simulink model "kepler_basic_2021b"  (R2021b)
settings: Solver=ode4  StartTime=0.0  StopTime=6000  FixedStep=0.01  RelTol=1e-3
(part 2 of 2)

== matlab function kepler_basic_2021b/[Mode3] Basic Kepler Propagate/MATLAB Function ==
  data: kepel input; statvec output
function statvec  = kepel_statvec (kepel)
%  [statvec] = kepel_statvec (kepel)
%	The function kepel_statvec transforms the keplerian
%	elements kepel into the corresponding state vector in
%	the same reference system.
%
% Input:
%	kepel
% 		vector containing the keplerian elements:
%		(1) - semimajor axis of the orbit in meters.
%		(2) - eccentricity.
%		(3) - inclinatsion in radians.
%		(4) - right ascension of ascending node in radians.
%		(5) - argument of perigee in radians.
%		(6) - mean anomaly in radians.
% Output:
%	statvec
%  		state vector in meters and meters/second.
%
% Authors:
%	Helio K. Kuga;
%	Valder M. Medeiros;
%	Valdemir Carrara		february/80		version 1.0
%	Valdemir Carrara		july 2005		(C version)
%   Valdemir Carrara            March/09        Matlab

EARTH_GRAVITY	= 3.9860064e+14;		% Earth's gravitational constant (m**3/s**2)

a    = kepel(1);	% semi-major axis
exc  = kepel(2);	% eccentricity

c1   = sqrt(1. - exc*exc);

%     rotation matrix

orb2iner = rotmaz(-kepel(4))*rotmax(-kepel(3))*rotmaz(-kepel(5));

%     Kepler's equation

E    = kepler(kepel(6), exc);

sE   = sin(E);
cE   = cos(E);
c3   = sqrt(EARTH_GRAVITY/a)/(1. - exc*cE);

%     state vector

statvec = [[a*(cE - exc), a*c1*sE, 0]*orb2iner', [-c3*sE, c1*c3*cE, 0]*orb2iner'];

end

function [rot_mat] = rotmax (angle)
% [rot_mat] = rotmax (angle)
%   To obtain the rotation matrix around the X axis given the
%   rotation angle.
% inputs:
%   angle
%       rotation angle, in radians.
% outputs:
%   rot_mat
%       rotation matrix (3, 3)
%

% Valdemir Carrara, Sep, 1998

coan    =  cos(angle);
sian    =  sin(angle);

rot_mat =  [1, 0, 0; 0, coan, sian; 0, -sian, coan];

end

function [rot_mat] = rotmay (angle)
% [rot_mat] = rotmay (angle)
%   To obtain the rotation matrix around the Y axis given the
%   rotation angle.
% inputs:
%   angle
%       rotation angle, in radians.
% outputs:
%   rot_mat
%       rotation matrix (3, 3)
%

% Valdemir Carrara, Sep, 1998


coan    =  cos(angle);
sian    =  sin(angle);

rot_mat =  [coan, 0, -sian; 0, 1, 0; sian, 0, coan];

end

function [rot_mat] = rotmaz (angle)
% [rot_mat] = rotmaz (angle)
%   To obtain the rotation matrix around the Z axis given the
%   rotation angle.
% inputs:
%   angle
%       rotation angle, in radians.
% outputs:
%   rot_mat
%       rotation matrix (3, 3)
%

% Valdemir Carrara, Sep, 1998

coan    =  cos(angle);
sian    =  sin(angle);

rot_mat =  [coan, sian, 0; -sian, coan, 0; 0, 0, 1];
end

function [eccentric] = kepler (mean_anomaly, eccentricity)
% [eccentric] = kepler (mean_anomaly, eccentricity)
%	The subroutine kepler finds a solution to the
%	kepler's equation.
%
% Input:
%	mean_anomaly
%		mean anomaly in radians.
%	eccentricity
%		eccentricity.
%
% Output:
%	eccentric
%		eccentric anomaly in radians.
%
% Authors:
%	Valder M. de Medeiros		june/81		version 2.0
%	Valdemir Carrara			july 2005	(C version)
%   Valdemir Carrara            March/09        Matlab

exc2    = eccentricity*eccentricity;
am1     = mod (mean_anomaly, 2*pi);
am2     = am1 + am1;
am3     = am1 + am2;
shoot   = am1 + eccentricity*(1. - 0.125*exc2)*sin(am1) + ...
		0.5*exc2*(sin(am2) + 0.75*eccentricity*sin(am3));
shoot   = mod (shoot, 2*pi);

e1      = 1.0;
ic      = 0;

while ((abs(e1) > 1.e-12) && (ic <= 10)) 
	e1    = (shoot - am1 - eccentricity*sin(shoot)) / ...
			(1.0 - eccentricity*cos(shoot));
    shoot = shoot - e1;
    ic    = ic + 1;
end

if (ic >= 10)
    disp ('warning ** subroutine kepler did not converge in 10 iterations');
end

eccentric = shoot;


end

== matlab function kepler_basic_2021b/[Mode4] Propat vs Kepler:Twobody Equation Integral Comparison/Kepler Propagate ==
  data: initial_condition input; dfdt output
function dfdt  = eq_propagate(initial_condition)
% Lectures_TwoBodyProblem.pdf
% 우주시스템입문 - 도미타 노부유키 eq(7.8) p136
% https://en.wikipedia.org/wiki/Standard_gravitational_parameter
u  = 3.9860064e+14; % earth gravitional parameter
Re = 6378137;      % earth radius [m]

dfdt = zeros(size(initial_condition));

% x=x
% x1=dx/dt
% dx1/dt = d^2(x)/dt

x1 = initial_condition(4); % x1 = dx/dt
y1 = initial_condition(5); % y1 = dy/dt
z1 = initial_condition(6); % z1 = dz/dt
x  = initial_condition(1); % x
y  = initial_condition(2); % y
z  = initial_condition(3); % z

r=sqrt(x^2+y^2+z^2);

% % %   Keplar Motion Equatnion
% % %  => r_dd + u/(r^3)r_ = 0 => r_dd = -u/(r^3)r_
dfdt(1) = x1;
dfdt(2) = y1;
dfdt(3) = z1;
dfdt(4) = -u*x/(r^3);
dfdt(5) = -u*y/(r^3);
dfdt(6) = -u*z/(r^3);

end

== matlab function kepler_basic_2021b/[Mode4] Propat vs Kepler:Twobody Equation Integral Comparison/MATLAB Function2 ==
  data: kepel input; statvec output
function statvec  = kepel_statvec (kepel)
%  [statvec] = kepel_statvec (kepel)
%	The function kepel_statvec transforms the keplerian
%	elements kepel into the corresponding state vector in
%	the same reference system.
%
% Input:
%	kepel
% 		vector containing the keplerian elements:
%		(1) - semimajor axis of the orbit in meters.
%		(2) - eccentricity.
%		(3) - inclinatsion in radians.
%		(4) - right ascension of ascending node in radians.
%		(5) - argument of perigee in radians.
%		(6) - mean anomaly in radians.
% Output:
%	statvec
%  		state vector in meters and meters/second.
%
% Authors:
%	Helio K. Kuga;
%	Valder M. Medeiros;
%	Valdemir Carrara		february/80		version 1.0
%	Valdemir Carrara		july 2005		(C version)
%   Valdemir Carrara            March/09        Matlab

EARTH_GRAVITY	= 3.9860064e+14;		% Earth's gravitational constant (m**3/s**2)

a    = kepel(1);	% semi-major axis
exc  = kepel(2);	% eccentricity

c1   = sqrt(1. - exc*exc);

%     rotation matrix

orb2iner = rotmaz(-kepel(4))*rotmax(-kepel(3))*rotmaz(-kepel(5));

%     Kepler's equation

E    = kepler(kepel(6), exc);

sE   = sin(E);
cE   = cos(E);
c3   = sqrt(EARTH_GRAVITY/a)/(1. - exc*cE);

%     state vector

statvec = [[a*(cE - exc), a*c1*sE, 0]*orb2iner', [-c3*sE, c1*c3*cE, 0]*orb2iner'];

end

function [rot_mat] = rotmax (angle)
% [rot_mat] = rotmax (angle)
%   To obtain the rotation matrix around the X axis given the
%   rotation angle.
% inputs:
%   angle
%       rotation angle, in radians.
% outputs:
%   rot_mat
%       rotation matrix (3, 3)
%

% Valdemir Carrara, Sep, 1998

coan    =  cos(angle);
sian    =  sin(angle);

rot_mat =  [1, 0, 0; 0, coan, sian; 0, -sian, coan];

end

function [rot_mat] = rotmay (angle)
% [rot_mat] = rotmay (angle)
%   To obtain the rotation matrix around the Y axis given the
%   rotation angle.
% inputs:
%   angle
%       rotation angle, in radians.
% outputs:
%   rot_mat
%       rotation matrix (3, 3)
%

% Valdemir Carrara, Sep, 1998


coan    =  cos(angle);
sian    =  sin(angle);

rot_mat =  [coan, 0, -sian; 0, 1, 0; sian, 0, coan];

end

function [rot_mat] = rotmaz (angle)
% [rot_mat] = rotmaz (angle)
%   To obtain the rotation matrix around the Z axis given the
%   rotation angle.
% inputs:
%   angle
%       rotation angle, in radians.
% outputs:
%   rot_mat
%       rotation matrix (3, 3)
%

% Valdemir Carrara, Sep, 1998

coan    =  cos(angle);
sian    =  sin(angle);

rot_mat =  [coan, sian, 0; -sian, coan, 0; 0, 0, 1];
end

function [eccentric] = kepler (mean_anomaly, eccentricity)
% [eccentric] = kepler (mean_anomaly, eccentricity)
%	The subroutine kepler finds a solution to the
%	kepler's equation.
%
% Input:
%	mean_anomaly
%		mean anomaly in radians.
%	eccentricity
%		eccentricity.
%
% Output:
%	eccentric
%		eccentric anomaly in radians.
%
% Authors:
%	Valder M. de Medeiros		june/81		version 2.0
%	Valdemir Carrara			july 2005	(C version)
%   Valdemir Carrara            March/09        Matlab

exc2    = eccentricity*eccentricity;
am1     = mod (mean_anomaly, 2*pi);
am2     = am1 + am1;
am3     = am1 + am2;
shoot   = am1 + eccentricity*(1. - 0.125*exc2)*sin(am1) + ...
		0.5*exc2*(sin(am2) + 0.75*eccentricity*sin(am3));
shoot   = mod (shoot, 2*pi);

e1      = 1.0;
ic      = 0;

while ((abs(e1) > 1.e-12) && (ic <= 10)) 
	e1    = (shoot - am1 - eccentricity*sin(shoot)) / ...
			(1.0 - eccentricity*cos(shoot));
    shoot = shoot - e1;
    ic    = ic + 1;
end

if (ic >= 10)
    disp ('warning ** subroutine kepler did not converge in 10 iterations');
end

eccentric = shoot;


end

== matlab function kepler_basic_2021b/[Mode4] Propat vs Kepler:Twobody Equation Integral Comparison/MATLAB Function ==
  data: kepel input; statvec output
function statvec  = kepel_statvec (kepel)
%  [statvec] = kepel_statvec (kepel)
%	The function kepel_statvec transforms the keplerian
%	elements kepel into the corresponding state vector in
%	the same reference system.
%
% Input:
%	kepel
% 		vector containing the keplerian elements:
%		(1) - semimajor axis of the orbit in meters.
%		(2) - eccentricity.
%		(3) - inclinatsion in radians.
%		(4) - right ascension of ascending node in radians.
%		(5) - argument of perigee in radians.
%		(6) - mean anomaly in radians.
% Output:
%	statvec
%  		state vector in meters and meters/second.
%
% Authors:
%	Helio K. Kuga;
%	Valder M. Medeiros;
%	Valdemir Carrara		february/80		version 1.0
%	Valdemir Carrara		july 2005		(C version)
%   Valdemir Carrara            March/09        Matlab

EARTH_GRAVITY	= 3.9860064e+14;		% Earth's gravitational constant (m**3/s**2)

a    = kepel(1);	% semi-major axis
exc  = kepel(2);	% eccentricity

c1   = sqrt(1. - exc*exc);

%     rotation matrix

orb2iner = rotmaz(-kepel(4))*rotmax(-kepel(3))*rotmaz(-kepel(5));

%     Kepler's equation

E    = kepler(kepel(6), exc);

sE   = sin(E);
cE   = cos(E);
c3   = sqrt(EARTH_GRAVITY/a)/(1. - exc*cE);

%     state vector

statvec = [[a*(cE - exc), a*c1*sE, 0]*orb2iner', [-c3*sE, c1*c3*cE, 0]*orb2iner'];

end

function [rot_mat] = rotmax (angle)
% [rot_mat] = rotmax (angle)
%   To obtain the rotation matrix around the X axis given the
%   rotation angle.
% inputs:
%   angle
%       rotation angle, in radians.
% outputs:
%   rot_mat
%       rotation matrix (3, 3)
%

% Valdemir Carrara, Sep, 1998

coan    =  cos(angle);
sian    =  sin(angle);

rot_mat =  [1, 0, 0; 0, coan, sian; 0, -sian, coan];

end

function [rot_mat] = rotmay (angle)
% [rot_mat] = rotmay (angle)
%   To obtain the rotation matrix around the Y axis given the
%   rotation angle.
% inputs:
%   angle
%       rotation angle, in radians.
% outputs:
%   rot_mat
%       rotation matrix (3, 3)
%

% Valdemir Carrara, Sep, 1998


coan    =  cos(angle);
sian    =  sin(angle);

rot_mat =  [coan, 0, -sian; 0, 1, 0; sian, 0, coan];

end

function [rot_mat] = rotmaz (angle)
% [rot_mat] = rotmaz (angle)
%   To obtain the rotation matrix around the Z axis given the
%   rotation angle.
% inputs:
%   angle
%       rotation angle, in radians.
% outputs:
%   rot_mat
%       rotation matrix (3, 3)
%

% Valdemir Carrara, Sep, 1998

coan    =  cos(angle);
sian    =  sin(angle);

rot_mat =  [coan, sian, 0; -sian, coan, 0; 0, 0, 1];
end

function [eccentric] = kepler (mean_anomaly, eccentricity)
% [eccentric] = kepler (mean_anomaly, eccentricity)
%	The subroutine kepler finds a solution to the
%	kepler's equation.
%
% Input:
%	mean_anomaly
%		mean anomaly in radians.
%	eccentricity
%		eccentricity.
%
% Output:
%	eccentric
%		eccentric anomaly in radians.
%
% Authors:
%	Valder M. de Medeiros		june/81		version 2.0
%	Valdemir Carrara			july 2005	(C version)
%   Valdemir Carrara            March/09        Matlab

exc2    = eccentricity*eccentricity;
am1     = mod (mean_anomaly, 2*pi);
am2     = am1 + am1;
am3     = am1 + am2;
shoot   = am1 + eccentricity*(1. - 0.125*exc2)*sin(am1) + ...
		0.5*exc2*(sin(am2) + 0.75*eccentricity*sin(am3));
shoot   = mod (shoot, 2*pi);

e1      = 1.0;
ic      = 0;

while ((abs(e1) > 1.e-12) && (ic <= 10)) 
	e1    = (shoot - am1 - eccentricity*sin(shoot)) / ...
			(1.0 - eccentricity*cos(shoot));
    shoot = shoot - e1;
    ic    = ic + 1;
end

if (ic >= 10)
    disp ('warning ** subroutine kepler did not converge in 10 iterations');
end

eccentric = shoot;


end

== matlab function kepler_basic_2021b/[MODE2] Propat : Kepler to Statevec using Only Mean Anomaly/MATLAB Function ==
  data: statv input; kepel output
function kepel  = statvec_kepel (statv)
% [kepel] = statvec_kepel (statv)
%
%	The function statvec_kepel transforms the state vector statv
%	into the corresponding keplerian elements in the
%	same reference system.
%
% Input:
%	statv
%		state vector in meters and meters/second.
%
% Output:
%	statvec_kepel
%		vector containing the keplerian elements:
%		(1) - semimajor axis of the orbit in meters.
%		(2) - eccentricity.
%		(3) - inclination in radians.
%		(4) - right ascension of ascending node in radians.
%		(5) - argument of perigee in radians.
%		(6) - mean anomaly in radians.
%
% Authors:
%	Helio K. Kuga
%    Valder M. Medeiros
%	Valdemir Carrara			february/80			version 1.0
%	Helio K. Kuga     			august/82           version 2.0
%	Ulisses T V Guedes 			december/95	 		version 2.1
%               - fix perigee procedure when orbit plane
%                  equal to equatorial plane
%	Valdemir Carrara 			july/05				(C version)
%   Valdemir Carrara            March/09        Matlab

EARTH_GRAVITY	= 3.9860064e+14;		% Earth's gravitational constant (m**3/s**2)

xp  = [statv(1) statv(2) statv(3)];
xv  = [statv(4) statv(5) statv(6)];
r      = sqrt(xp*xp');
vq     = xv*xv';
ainv   = 2.0/r - vq/EARTH_GRAVITY;

h      = cross(xp, xv);
hm     = sqrt(h*h');
an = [0 0 0];
if (hm < 1.e-10)
    disp (' *** Message from function statvec_kepel: *** ');
    disp (' There are no keplerian elements corresponding to this state vector');
    kepel = [0, 0, 0, 0, 0, 0];
else
    h      = h/hm;
    incl   = acos(h(3));
    raan   = atan2(h(1), -h(2));
    d      = xp*xv' / EARTH_GRAVITY;
    esene  = d * sqrt(EARTH_GRAVITY*ainv);
    ecose  = 1 - r*ainv;
    exc    = sqrt(esene*esene + ecose*ecose);
    E      = atan2(esene, ecose);
    mean   = mod (E - esene, 2*pi);
    if mean < 0
        mean = mean + 2*pi;
    end

    if exc < 1.e-10
        arpe = 0;
    else
        dp     = 1./r - ainv;
        ev     = dp*xp - d*xv;
        abev   = sqrt(ev*ev');
        ev     = ev/abev;
        an(1)  = cos(raan);
        an(2)  = sin(raan);
        an(3)  = 0;
        fi     = ev*cross(h, an)';
        arpe = acos(ev*an');
        if fi < 0
            arpe  =  -arpe + 2*pi;
        end
    end

    kepel = [1./ainv, exc, incl, raan, arpe, mean];
end

end

== matlab function kepler_basic_2021b/[Mode3] Basic Kepler Propagate/MATLAB Function5 ==
  settings: updateMethod=DISCRETE
  data: statv input; kepel output
function kepel  = statvec_kepel (statv)
%	The function statvec_kepel transforms the state vector statv
%	into the corresponding keplerian elements in the
%	same reference system.
%
% Input:
%	statv
%		state vector in meters and meters/second.
%
% Output:
%	statvec_kepel
%		vector containing the keplerian elements:
%		(1) - semimajor axis of the orbit in meters.
%		(2) - eccentricity.
%		(3) - inclination in radians.
%		(4) - right ascension of ascending node in radians.
%		(5) - argument of perigee in radians.
%		(6) - mean anomaly in radians.

EARTH_GRAVITY	= 3.9860064e+14;		% Earth's gravitational constant (m**3/s**2)

    xp     = [statv(1),statv(2),statv(3)];
    xv     = [statv(4),statv(5),statv(6)];
    r      = sqrt(xp*xp');
    vq     = xv*xv';
    ainv   = 2.0/(r) - vq/EARTH_GRAVITY;

    h      = cross(xp, xv);
    hm     = sqrt(h*h');
    if (hm < 1.e-10)
        disp (' *** Message from function statvec_kepel: *** ');
        disp (' There are no keplerian elements corresponding to this state vector');
        kepel = [0, 0, 0, 0, 0, 0];
    else
        h      = h/hm;
        incl   = acos(h(3));
        raan   = atan2(h(1), -h(2));
        d      = xp*xv' / EARTH_GRAVITY;
        esene  = d * sqrt(EARTH_GRAVITY*ainv);
        ecose  = 1 - r*ainv;
        exc    = sqrt(esene*esene + ecose*ecose);
        E      = atan2(esene, ecose);
        mean   = mod (E - esene, 2*pi);
        an = [0 0 0];
        if mean < 0
            mean = mean + 2*pi;
        end
        if exc < 1.e-10
            arpe = 0;
        else
            dp     = 1./r - ainv;
            ev     = dp*xp - d*xv;
            abev   = sqrt(ev*ev');
            ev     = ev/abev;
            an(1)  = cos(raan);
            an(2)  = sin(raan);
            an(3)  = 0;
            fi     = ev*cross(h, an)';
            arpe = acos(ev*an');
            if fi < 0
                arpe  =  -arpe + 2*pi;
            end
        end

        kepel = [(1./ainv), exc, incl, raan, arpe, mean];
    end



end

== matlab function kepler_basic_2021b/[Mode4] Propat vs Kepler:Twobody Equation Integral Comparison/Propat Propagator No J2&J4/Keplerian Differential Equation ==
  data: kepel input; deltakep output
function deltakep  = delkep(kepel)
% [deltakep] = delkep (kep_el)
%	Function delkep calculates the rate of
%	variation of keplerian elements, considering only
%	J2 and J4.
%
% Input:
%	kep_el
% 		vector with the keplerian elements:
%		(1) - semimajor axis of the orbit in meters.
%		(2) - eccentricity.
%		(3) - inclination in radians.
%		(4) - right ascension of ascending node in radians.
%		(5) - argument of perigee in radians.
%		(6) - mean anomaly in radians.
%       Obs: 4,5 and 6 are not used
%
% Output:
%	deltakep
%		(1) = 0
%		(2) = 0
%		(3) = 0
%		(4) - variation rate of the right ascension of
%		      ascending node, in radians/second.
%		(5) - variation rate of the argument of perigee,
%			  in radians/second.
%		(6) - variation rate of the mean anomaly, in
%			  radians/second.
%
% Authors:
%	Valder M. de Medeiros  	september/81 	version 1.0
%	Valdemir Carrara 		july 2005		(C Version)
%   Valdemir Carrara            March/09        Matlab

EARTH_RADIUS	= 6378139.;				% Earth's radius in meters
EARTH_GRAVITY	= 3.9860064e+14;		% Earth's gravitational constant (m**3/s**2)
% J_2 			=  1.0826268362e-3;		% = 484.16544e-6 * SQRT(5.e0)
% J_4 			= -1.62336e-6;			% = -0.54112e-6 * 3e0
J_2 			=  0;		% = 484.16544e-6 * SQRT(5.e0)
J_4 			=  0;			% = -0.54112e-6 * 3e0

seix = kepel(1);
exce = kepel(2);
exc2 = exce*exce;
eta2 = 1. - exc2;
eta1 = sqrt(eta2);
teta = cos(kepel(3));
tet2 = teta*teta;
tet4 = tet2*tet2;
aux0 = sqrt(EARTH_GRAVITY/(seix*seix*seix));
plar = EARTH_RADIUS/(seix*eta2);
pla2 = plar*plar;
gam2 = 0.5*J_2*pla2;
gam4 = -0.375*J_4*pla2*pla2;

deltakep = [0, 0, 0, 0, 0, 0];

deltakep(4) = aux0*teta*(3.*gam2*(-1. + 0.125*gam2*(9.*eta2 + 12.*eta1 - ...
	   5. - (5.*eta2 + 36.*eta1 + 35.)*tet2)) + ...
	   1.25*gam4*(5. - 3.*eta2)*(3. - 7.*tet2));
deltakep(5) = aux0*(1.5*gam2*((5.*tet2 - 1.) + ...
	   0.0625*gam2*(25.*eta2 + 24.*eta1 - ...
	   35. + (90. - 192.*eta1 - 126.*eta2)*tet2 + ...
	   (385. + 360.*eta1 + 45.*eta2)*tet4)) + ...
	   0.3125*gam4*(21. - 9.*eta2 + (-270. + 126.*eta2)*tet2 + ...
	   (385. - 189.*eta2)*tet4));
deltakep(6) = aux0*(1. + eta1*(1.5*gam2*((3.*tet2 - 1.) + ...
	   0.0625*gam2*(16.*eta1 + 25.*eta2 - 15. + ...
	   (30. - 96.*eta1 - 90.*eta2)*tet2 + ...
	   (105. + 144.*eta1 + 25.*eta2)*tet4)) + ...
	   0.9375*gam4*exc2*(3. - 30.*tet2 + 35.*tet4)));

end
